simulink library "PuppyLibrary"  (R2021b)
settings: Solver=VariableStepAuto  StartTime=0.0  StopTime=10.0  RelTol=1e-3
libraries: embedlinuxBasiclib x5, raspberrypiCommlib x2
settings Model: Creator=kboxi  LastModifiedBy=MSI-NB
settings SolverCC: AlgebraicLoopSolver=TrustRegion
settings DebuggingCC: SFMachineParentedDataDiag=warning

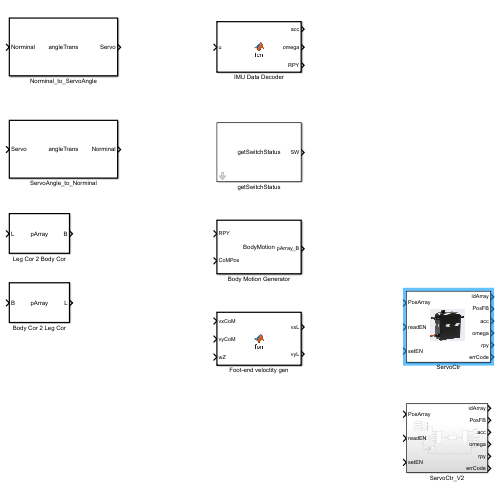
[thumbnail: Simulink's stored preview of the top-level diagram]
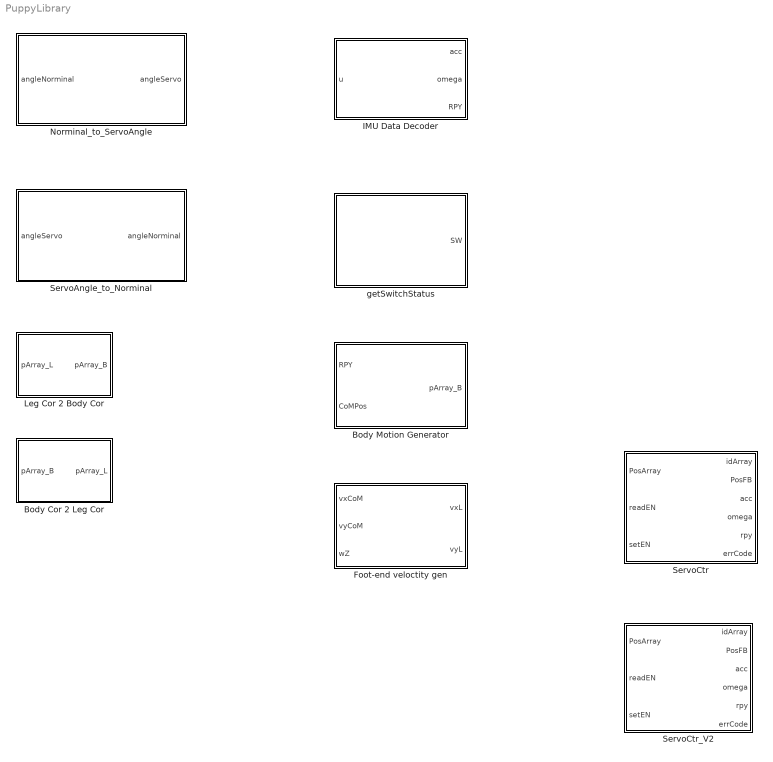
== system PuppyLibrary ==
  Body Cor 2 Leg Cor : MATLAB Function  TreatAsAtomicUnit=on
  Body Motion Generator : MATLAB Function  TreatAsAtomicUnit=on
  Foot-end veloctity gen : MATLAB Function  TreatAsAtomicUnit=on
  IMU Data Decoder : MATLAB Function  TreatAsAtomicUnit=on
  Leg Cor 2 Body Cor : MATLAB Function  TreatAsAtomicUnit=on
  Norminal_to_ServoAngle : MATLAB Function  TreatAsAtomicUnit=on
  ServoAngle_to_Norminal : MATLAB Function  TreatAsAtomicUnit=on
  ServoCtr : Subsystem
      mask Display: image('$imagefile'); % Use "Edit Image" on toolstrip to change.
  ServoCtr_V2 : Subsystem
  getSwitchStatus : Subsystem  mask{sampleTime=0.005}
      mask prompts: sampleTime "Sample Time"
      mask help: Read foot-end switch values
      mask Display: disp('getSwitchStatus')

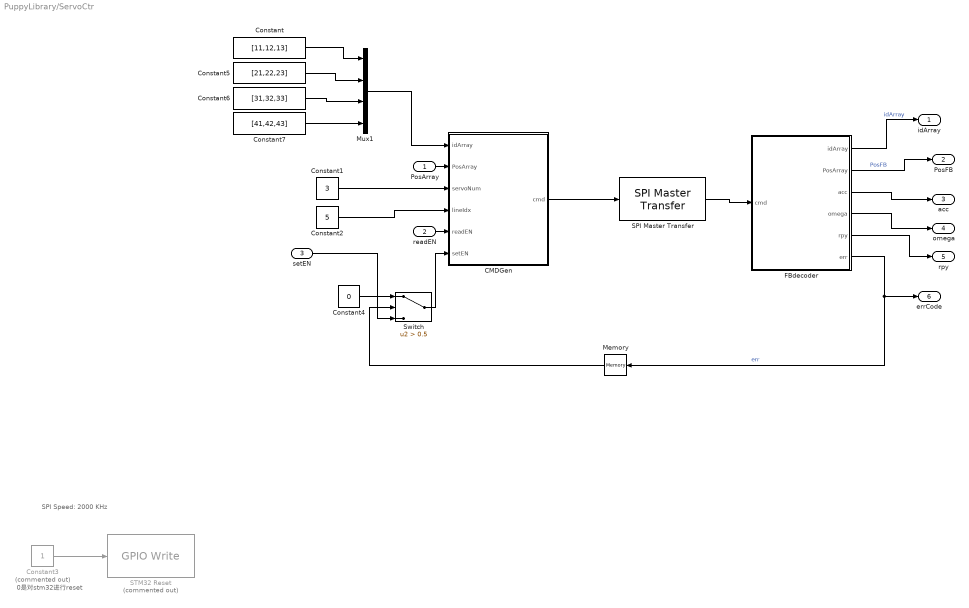
== system PuppyLibrary/ServoCtr ==
  note: SPI Speed: 2000 KHz
  note: 0是对stm32进行reset
  PosArray : Inport
  readEN : Inport  Port=2
  setEN : Inport  Port=3
  CMDGen : MATLAB Function  TreatAsAtomicUnit=on
  Constant : Constant  Value=[11,12,13]
  Constant1 : Constant  Value=3
  Constant2 : Constant  Value=5
  Constant3 : Constant  Commented=on
  Constant4 : Constant  Value=0
  Constant5 : Constant  Value=[21,22,23]
  Constant6 : Constant  Value=[31,32,33]
  Constant7 : Constant  Value=[41,42,43]
  FBdecoder : MATLAB Function  TreatAsAtomicUnit=on
  Memory : Memory  InitialCondition=1
  Mux1 : Mux
  SPI Master Transfer : raspberrypiCommlib/SPI Master Transfer  BoardProperty=Pi 4 Model B  SSPin=SPI0_CE0  SPIModule=uint32(0)  Mode=Master  BusSpeed=1000000  Pin=uint32(0)  FirstBitToTransfer=Most significant bit (MSB)  ClockMode=0  BlockFunction=Transfer  RegisterAddress=0  OutputDataType=int8  OutputDataLength=1
      settings: SourceProductBaseCode=RASPPI
  STM32 Reset : embedlinuxBasiclib/GPIO Write  Commented=on  board=Pi 4 Model B  gpio=23  direction=Output  blockPlatform=Raspberry Pi
      settings: SourceProductBaseCode=SC_BEAGLEBONE_BLUE,EMBEDDEDLINUX,NVIDIA,RASPPIIO
  Switch : Switch  Criteria=u2 > Threshold  Threshold=0.5
  idArray : Outport
  PosFB : Outport  Port=2
  acc : Outport  Port=3
  omega : Outport  Port=4
  rpy : Outport  Port=5
  errCode : Outport  Port=6
  wires:
  Constant5/1 -> Mux1/2
  FBdecoder/2(PosArray) -> PosFB/1  "PosFB"
  FBdecoder/1(idArray) -> idArray/1  "idArray"
  Constant7/1 -> Mux1/4
  readEN/1 -> CMDGen/5(readEN)
  Constant6/1 -> Mux1/3
  CMDGen/1(cmd) -> SPI Master Transfer/1
  Constant/1 -> Mux1/1
  FBdecoder/6(err) -> Memory/1, errCode/1  "err"
  Mux1/1 -> CMDGen/1(idArray)
  Constant1/1 -> CMDGen/3(servoNum)
  Constant2/1 -> CMDGen/4(lineIdx)
  PosArray/1 -> CMDGen/2(PosArray)
  Constant3/1 -> STM32 Reset/1
  FBdecoder/3(acc) -> acc/1
  FBdecoder/4(omega) -> omega/1
  FBdecoder/5(rpy) -> rpy/1
  Memory/1 -> Switch/2
  Constant4/1 -> Switch/1
  setEN/1 -> Switch/3
  Switch/1 -> CMDGen/6(setEN)
  SPI Master Transfer/1 -> FBdecoder/1(cmd)

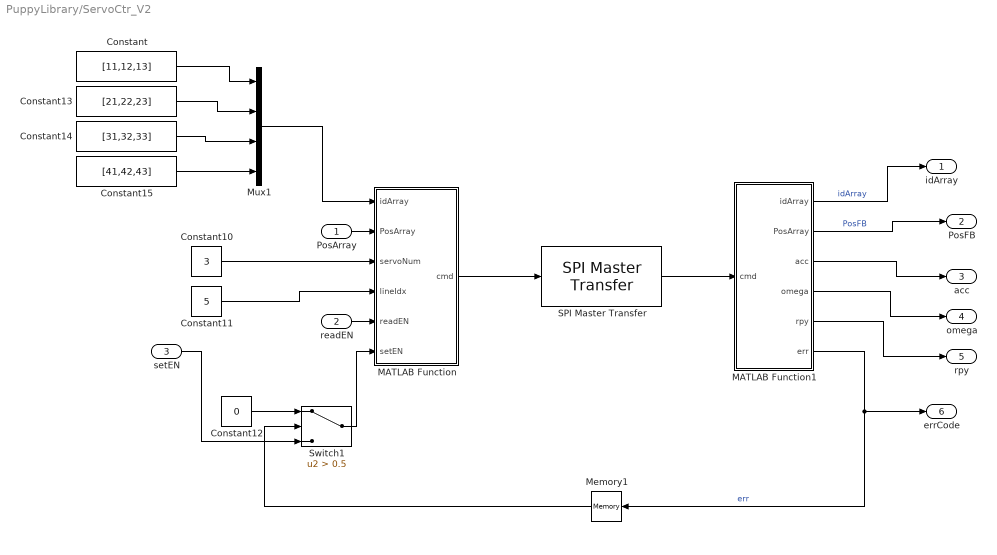
== system PuppyLibrary/ServoCtr_V2 ==
  PosArray : Inport
  readEN : Inport  Port=2
  setEN : Inport  Port=3
  Constant : Constant  Value=[11,12,13]
  Constant10 : Constant  Value=3
  Constant11 : Constant  Value=5
  Constant12 : Constant  Value=0
  Constant13 : Constant  Value=[21,22,23]
  Constant14 : Constant  Value=[31,32,33]
  Constant15 : Constant  Value=[41,42,43]
  MATLAB Function : MATLAB Function  TreatAsAtomicUnit=on
  MATLAB Function1 : MATLAB Function  TreatAsAtomicUnit=on
  Memory1 : Memory  InitialCondition=1
  Mux1 : Mux
  SPI Master Transfer : raspberrypiCommlib/SPI Master Transfer  BoardProperty=Pi 4 Model B  SSPin=SPI0_CE0  SPIModule=uint32(0)  Mode=Master  BusSpeed=1000000  Pin=uint32(0)  FirstBitToTransfer=Most significant bit (MSB)  ClockMode=0  BlockFunction=Transfer  RegisterAddress=0  OutputDataType=int8  OutputDataLength=1
      settings: SourceProductBaseCode=RASPPI
  Switch1 : Switch  Criteria=u2 > Threshold  Threshold=0.5
  idArray : Outport
  PosFB : Outport  Port=2
  acc : Outport  Port=3
  omega : Outport  Port=4
  rpy : Outport  Port=5
  errCode : Outport  Port=6
  wires:
  MATLAB Function1/5(rpy) -> rpy/1
  MATLAB Function1/3(acc) -> acc/1
  MATLAB Function1/4(omega) -> omega/1
  Constant15/1 -> Mux1/4
  Constant12/1 -> Switch1/1
  MATLAB Function1/2(PosArray) -> PosFB/1  "PosFB"
  MATLAB Function1/1(idArray) -> idArray/1  "idArray"
  SPI Master Transfer/1 -> MATLAB Function1/1(cmd)
  MATLAB Function1/6(err) -> errCode/1, Memory1/1  "err"
  setEN/1 -> Switch1/3
  Constant14/1 -> Mux1/3
  Memory1/1 -> Switch1/2
  Constant/1 -> Mux1/1
  Constant13/1 -> Mux1/2
  MATLAB Function/1(cmd) -> SPI Master Transfer/1
  Mux1/1 -> MATLAB Function/1(idArray)
  Switch1/1 -> MATLAB Function/6(setEN)
  Constant10/1 -> MATLAB Function/3(servoNum)
  Constant11/1 -> MATLAB Function/4(lineIdx)
  PosArray/1 -> MATLAB Function/2(PosArray)
  readEN/1 -> MATLAB Function/5(readEN)

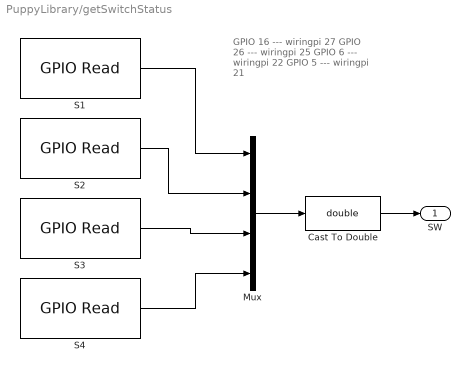
== system PuppyLibrary/getSwitchStatus ==
  note: GPIO 16 --- wiringpi 27
      | GPIO  26 --- wiringpi 25
      | GPIO 6 --- wiringpi 22
      | GPIO 5 --- wiringpi 21
  Cast To Double : DataTypeConversion  OutDataTypeStr=double
  Mux : Mux
  S1 : embedlinuxBasiclib/GPIO Read  board=Pi 4 Model B  gpio=24  internalResistor=Off  sampleTime=sampleTime  direction=Input  blockPlatform=Raspberry Pi
      settings: SourceProductBaseCode=SC_BEAGLEBONE_BLUE,EMBEDDEDLINUX,NVIDIA,RASPPIIO
  S2 : embedlinuxBasiclib/GPIO Read  board=Pi 4 Model B  gpio=23  internalResistor=Off  sampleTime=sampleTime  direction=Input  blockPlatform=Raspberry Pi
      settings: SourceProductBaseCode=SC_BEAGLEBONE_BLUE,EMBEDDEDLINUX,NVIDIA,RASPPIIO
  S3 : embedlinuxBasiclib/GPIO Read  board=Pi 4 Model B  gpio=18  internalResistor=Off  sampleTime=sampleTime  direction=Input  blockPlatform=Raspberry Pi
      settings: SourceProductBaseCode=SC_BEAGLEBONE_BLUE,EMBEDDEDLINUX,NVIDIA,RASPPIIO
  S4 : embedlinuxBasiclib/GPIO Read  board=Pi 4 Model B  gpio=4  internalResistor=Off  sampleTime=sampleTime  direction=Input  blockPlatform=Raspberry Pi
      settings: SourceProductBaseCode=SC_BEAGLEBONE_BLUE,EMBEDDEDLINUX,NVIDIA,RASPPIIO
  SW : Outport  OutDataTypeStr=double  PortDimensions=[4,1]
  wires:
  S4/1 -> Mux/4
  S2/1 -> Mux/2
  S3/1 -> Mux/3
  S1/1 -> Mux/1
  Mux/1 -> Cast To Double/1
  Cast To Double/1 -> SW/1

== matlab function PuppyLibrary/ServoCtr_V2/MATLAB Function1 ==
  data: cmd input uint8 size=[60 1]; idArray output; PosArray output; acc output; omega output; rpy output; err output
function [idArray,PosArray,acc,omega,rpy,err] = fcn(cmd)
err=0;
if uint8(cmd(1))~=0x66
    err=1;
end
check=mod(sum(uint16(cmd(1:59))),256);
if uint8(check)~=cmd(60)
    err=1;
end
servoNum=cmd(2);
idArray=zeros(12,1);
PosArray=zeros(12,1);
for i=1:1:12
    idArray(i)=cmd(2+i);
    idxPos=15+i*2-2;
    temp=typecast(cmd(idxPos:idxPos+1),'int16');
    PosArray(i)=double(temp)/10;
end
acc=zeros(3,1);
for i=1:1:3
    acc(i)=double(typecast(cmd(39+i*2-2:39+i*2-1),'int16'))/32768*16*9.8;
end
omega=zeros(3,1);
for i=1:1:3
    omega(i)=double(typecast(cmd(45+i*2-2:45+i*2-1),'int16'))/32768*2000/180*pi;
end
rpy=zeros(3,1);
for i=1:1:3
    rpy(i)=double(typecast(cmd(51+i*2-2:51+i*2-1),'int16'))/32768*180/180*pi;
end

== matlab function PuppyLibrary/ServoAngle_to_Norminal ==
  data: angleServo input; angleNorminal output
function angleNorminal = fcn(angleServo)
% PuppyLibrary API
% transform servo feedback angles to norminal format for FK

% angleServo: [12,1] vector, output to servos, labels should be [11,12,13,...,41,42,43]
% clock-wise position rotation, unit is degree
% angleNorminal: [12,1] vector, unit is radiuns, counter clock-wise
% rotation
%angleOff=[-8.996;-0.7468;-7.452;-7.073;-1.056;4.301;3.073;5.056;6.301;1.877;-5.857;2]; % 2021-8-23
angleOff=[-7.494;0.4002;-7.452;-7.073;-1.056;4.301;3.073;5.056;6.301;3.35;-4.745;2]; %2021/12/11
angleNorminal = (angleServo-angleOff)/180*pi;
angleNorminal(9)=-angleNorminal(9);
angleNorminal(12)=-angleNorminal(12);
% for current servos, clock-wise rotation is the position direction
angleNorminal=-angleNorminal;

== matlab function PuppyLibrary/Norminal_to_ServoAngle ==
  data: angleNorminal input; angleServo output
function angleServo = fcn(angleNorminal)
% PuppyLibrary API
% transform IK's results to servo commands

% angleNorminal: [12,1] vector, unit is radiuns, 
% counter clock-wise rotation, results direct from IK.
% angleServo: [12,1] vector, output to servos, labels should be [11,12,13,...,41,42,43]
% clock-wise position rotation, unit is degree
%angleOff=[-8.996;-0.7468;-7.452;-7.073;-1.056;4.301;3.073;5.056;6.301;1.877;-5.857;2]; % 2021-8-23
angleOff=[-7.494;0.4002;-7.452;-7.073;-1.056;4.301;3.073;5.056;6.301;3.35;-4.745;2]; %2021/12/11

angleServo = angleNorminal/pi*180;
angleServo(9)=-angleServo(9);
angleServo(12)=-angleServo(12);
% for current servos, clock-wise rotation is the position direction
angleServo=-angleServo;
angleServo=angleServo+angleOff;

== matlab function PuppyLibrary/IMU Data Decoder ==
  data: u input; acc output size=[3 1]; omega output size=[3 1]; RPY output size=[3 1]
function [acc,omega,RPY] = fcn(u)
% register order must be [0x34 0x35 0x36 0x37 0x38 0x39 0x3d 0x3e 0x3f]
% the output acc is the decoupled linear acc
% acc and omega is in the imu coordinate
% omega is in radian
u=reshape(u,9,1);
acc=double(typecast(u(1:3),'int16'))/32768*4*9.8; % 4g is the range
omega=double(typecast(u(4:6),'int16'))/32768*1000; % 1000 is the range
RPY=double(typecast(u(7:9),'int16'))/32768*180/180*pi;
acc=acc+[0;0;0];
Rx=[1,0,0;
    0,cos(RPY(1)),-sin(RPY(1));
    0,sin(RPY(1)),cos(RPY(1))];
Ry=[cos(RPY(2)),0,sin(RPY(2));
    0,1,0;
    -sin(RPY(2)),0,cos(RPY(2))];
Rz=[cos(RPY(3)),-sin(RPY(3)),0;
    sin(RPY(3)),cos(RPY(3)),0;
    0,0,1];
Gnow=(Rz*Ry*Rx)'*[0;0;-9.8];
acc=acc+Gnow;

== matlab function PuppyLibrary/Leg Cor 2 Body Cor ==
  data: pArray_L input size=[12,1]; pArray_B output size=[12,1]
function pArray_B = fcn(pArray_L)
% transform foot-end pos from leg coordinate to body coordinate
yWidth=97; % distantce between left and right roll axis, i.e. distance between left and right leg coordinates
xWidth=210.8; % distance between fore and hind pitch axis, i.e. distance between fore and hind leg coordinates
piOFF=zeros(12,1);
piOFF(1:3)=[xWidth;yWidth;0]/2;
piOFF(4:6)=[xWidth;-yWidth;0]/2;
piOFF(7:9)=[-xWidth;yWidth;0]/2;
piOFF(10:12)=[-xWidth;-yWidth;0]/2;
pArray_B=pArray_L+piOFF;

== matlab function PuppyLibrary/Body Cor 2 Leg Cor ==
  data: pArray_B input size=[12,1]; pArray_L output size=[12,1]
function pArray_L = fcn(pArray_B)
% transform foot-end pos from leg coordinate to body coordinate
yWidth=97; % distantce between left and right roll axis, i.e. distance between left and right leg coordinates
xWidth=210.8; % distance between fore and hind pitch axis, i.e. distance between fore and hind leg coordinates
piOFF=zeros(12,1);
piOFF(1:3)=[xWidth;yWidth;0]/2;
piOFF(4:6)=[xWidth;-yWidth;0]/2;
piOFF(7:9)=[-xWidth;yWidth;0]/2;
piOFF(10:12)=[-xWidth;-yWidth;0]/2;
pArray_L=pArray_B-piOFF;

== matlab function PuppyLibrary/Body Motion Generator ==
  data: RPY input; pArray_B output size=[12 1]; CoMPos input
function pArray_B = fcn(RPY, CoMPos)
% CoMPos are in mm
tempParray_B=zeros(12,1);
yWidth=97; % distantce between left and right roll axis, i.e. distance between left and right leg coordinates
xWidth=210.8; % distance between fore and hind pitch axis, i.e. distance between fore and hind leg coordinates
piOFF=zeros(12,1);
piOFF(1:3)=[xWidth;yWidth;0]/2;
piOFF(4:6)=[xWidth;-yWidth;0]/2;
piOFF(7:9)=[-xWidth;yWidth;0]/2;
piOFF(10:12)=[-xWidth;-yWidth;0]/2;
tempParray_B=tempParray_B+piOFF+[0;37;0;0;-37;0;0;37;0;0;-37;0];

Ry=[cos(RPY(2)),0,sin(RPY(2));
    0,1,0;
    -sin(RPY(2)),0,cos(RPY(2))];
Rx=[1,0,0;
    0,cos(RPY(1)),-sin(RPY(1));
    0,sin(RPY(1)),cos(RPY(1))];
Rz=[cos(RPY(3)),-sin(RPY(3)),0;
    sin(RPY(3)),cos(RPY(3)),0;
    0,0,1];
R=Rz*Ry*Rx;
tmppArray_B=R'*reshape(tempParray_B,3,4)-[CoMPos(1);CoMPos(2);CoMPos(3)]*[1,1,1,1];
tmppArray_B=reshape(tmppArray_B,12,1);
pArray_B=zeros(12,1);
pArray_B(:,1)=tmppArray_B;

== matlab function PuppyLibrary/Foot-end veloctity gen ==
  data: vxCoM input; vxL output; vyCoM input; vyL output; wZ input
function [vxL,vyL] = fcn(vxCoM,vyCoM,wZ)
tempParray_B=zeros(12,1);
yWidth=97; % distantce between left and right roll axis, i.e. distance between left and right leg coordinates
xWidth=210.8; % distance between fore and hind pitch axis, i.e. distance between fore and hind leg coordinates
piOFF=zeros(12,1);
piOFF(1:3)=[xWidth;yWidth;0]/2;
piOFF(4:6)=[xWidth;-yWidth;0]/2;
piOFF(7:9)=[-xWidth;yWidth;0]/2;
piOFF(10:12)=[-xWidth;-yWidth;0]/2;
tempParray_B=tempParray_B+piOFF+[0;37;0;0;-37;0;0;37;0;0;-37;0];

wZ=-wZ;
wZcap=[0,-wZ,0;
    wZ,0,0;
    0,0,0];
vL=wZcap*reshape(tempParray_B,3,4)-vxCoM*[ones(1,4);zeros(2,4)]-vyCoM*[zeros(1,4);ones(1,4);zeros(1,4)];
vxL=vL(1,:);
vyL=vL(2,:);

== matlab function PuppyLibrary/ServoCtr/CMDGen ==
  data: idArray input; cmd output size=[60 1]; PosArray input; servoNum input; lineIdx input; readEN input; setEN input
function cmd = fcn(idArray,PosArray,servoNum,lineIdx,readEN,setEN)
% length of idArray must not exceed 12!
cmd=uint8(zeros(60,1));
cmd(1)=0x66;
cmd(2)=servoNum;

if readEN>0.5 && setEN>0.5
    cmd(3)=2;
elseif readEN>0.5 && setEN<0.5
    cmd(3)=0;
elseif readEN<0.5 && setEN>0.5
    cmd(3)=1;
else
    cmd(3)=3;
end
lineIdx=uint8(lineIdx);
cmd(3)=cmd(3)+lineIdx*10;

for i=1:1:length(idArray)
    cmd(4+i-1)=idArray(i);
    sendAngle=int16(PosArray(i)*10);
    resAngle=typecast(sendAngle,'uint8');
    cmd(16+i*2-2)=resAngle(1);
    cmd(16+i*2-1)=resAngle(2);
end
cmd(60)=mod(sum(uint16(cmd(1:59))),256);

== matlab function PuppyLibrary/ServoCtr/FBdecoder ==
  data: cmd input size=[60 1]; idArray output; PosArray output; acc output; omega output; rpy output; err output
function [idArray,PosArray,acc,omega,rpy,err] = fcn(cmd)
err=0;
if uint8(cmd(1))~=0x66
    err=1;
end
check=mod(sum(uint16(cmd(1:59))),256);
if uint8(check)~=cmd(60)
    err=1;
end
servoNum=cmd(2);
idArray=zeros(12,1);
PosArray=zeros(12,1);
for i=1:1:12
    idArray(i)=cmd(2+i);
    idxPos=15+i*2-2;
    temp=typecast(cmd(idxPos:idxPos+1),'int16');
    PosArray(i)=double(temp)/10;
end
acc=zeros(3,1);
for i=1:1:3
    acc(i)=double(typecast(cmd(39+i*2-2:39+i*2-1),'int16'))/32768*16*9.8;
end
omega=zeros(3,1);
for i=1:1:3
    omega(i)=double(typecast(cmd(45+i*2-2:45+i*2-1),'int16'))/32768*2000/180*pi;
end
rpy=zeros(3,1);
for i=1:1:3
    rpy(i)=double(typecast(cmd(51+i*2-2:51+i*2-1),'int16'))/32768*180/180*pi;
end

== matlab function PuppyLibrary/ServoCtr_V2/MATLAB Function ==
  data: idArray input; cmd output uint8 size=[60 1]; PosArray input; servoNum input; lineIdx input; readEN input; setEN input
function cmd = fcn(idArray,PosArray,servoNum,lineIdx,readEN,setEN)
% length of idArray must not exceed 12!
cmd=uint8(zeros(60,1));
cmd(1)=0x66;
cmd(2)=servoNum;

if readEN>0.5 && setEN>0.5
    cmd(3)=2;
elseif readEN>0.5 && setEN<0.5
    cmd(3)=0;
elseif readEN<0.5 && setEN>0.5
    cmd(3)=1;
else
    cmd(3)=3;
end
lineIdx=uint8(lineIdx);
cmd(3)=cmd(3)+lineIdx*10;

for i=1:1:length(idArray)
    cmd(4+i-1)=idArray(i);
    sendAngle=int16(PosArray(i)*10);
    resAngle=typecast(sendAngle,'uint8');
    cmd(16+i*2-2)=resAngle(1);
    cmd(16+i*2-1)=resAngle(2);
end
cmd(60)=mod(sum(uint16(cmd(1:59))),256);
